simulink model "quad_with_sensor_fusion_discrete"  (R2022b)
settings: Solver=FixedStepDiscrete  StartTime=0.0  StopTime=120  FixedStep=0.005  RelTol=1e-3
values from neighbouring files (symbols this model uses):
  Ixc = 9373.661914436/1e6    (= 0.00937366191444)    [ParamsInit_test.m]
  Iyc = 11755.067703159/1e6    (= 0.0117550677032)    [ParamsInit_test.m]
  Izc = 17533.553367555/1e6    (= 0.0175335533676)    [ParamsInit_test.m]
  kd_h = damp_ratio_h*2*sqrt(kp_h*Vehicle.Airframe.mass)    [ParamsInit_test.m]
  kd_phi = damp_ratio_phi*2*sqrt(kp_phi*Ixc)    [ParamsInit_test.m]
  kd_theta = damp_ratio_theta*2*sqrt(kp_theta*Iyc)    [ParamsInit_test.m]
  kd_yaw = damp_ratio_yaw*2*sqrt(kp_yaw*Izc)    [ParamsInit_test.m]
  kp_h = omega_n_h^2*Vehicle.Airframe.mass    [ParamsInit_test.m]
  kp_phi = omega_n_phi^2*Ixc    (= 0.937366191444)    [ParamsInit_test.m]
  kp_position = 0.1    [ParamsInit_test.m]
  kp_theta = omega_n_theta^2*Iyc    (= 1.17550677032)    [ParamsInit_test.m]
  kp_vx = 0.25    [ParamsInit_test.m]
  kp_vy = 0.25    [ParamsInit_test.m]
  kp_yaw = omega_n_yaw^2*Izc    (= 0.0175335533676)    [ParamsInit_test.m]
undefined symbols (not defined in the file or in its folder): DiscIntNeverNeededParam, Vehicle
libraries: simulink x3, aerolibconvert2 x2, mspfiltlib x1, sensorinslib x1, aerolibasang x1, sharedtransform x1, mspsensorlib x1, sensorgpslib x1, aerolibanimutils x1, uavutilslib x1
(part 2 of 2)

== matlab function quad_with_sensor_fusion_discrete/Sensors and Sensor Fusion/MATLAB Function1 ==
  data: u input; y output
function y = fcn(u)

y = zeros(3,3);

a = u(1);
b = u(2);
c = u(3);

y(1,1) = cos(b)*cos(c);
y(1,2) = cos(b)*sin(c);
y(1,3) = -sin(b);
y(2,1) = sin(a)*sin(b)*cos(c)-cos(a)*sin(c);
y(2,2) = sin(a)*sin(b)*sin(c)+cos(a)*cos(c);
y(2,3) = sin(a)*cos(b);
y(3,1) = cos(a)*sin(b)*cos(c)+sin(a)*sin(c);
y(3,2) = cos(a)*sin(b)*sin(c)-sin(a)*cos(c);
y(3,3) = cos(a)*cos(b);

end

== matlab function quad_with_sensor_fusion_discrete/Plant(UAV EOM)(Non-linear)/6DOF CORE/Subsystem10/Subsystem/MATLAB Function ==
  data: m input; udot output; Fx input; V input; W input; Q input; R input
function udot = fcn(m,Fx,V,W,Q,R)
    udot = Fx/m+R*V-Q*W;
end

== matlab function quad_with_sensor_fusion_discrete/Plant(UAV EOM)(Non-linear)/6DOF CORE/Subsystem10/Subsystem1/MATLAB Function ==
  data: m input; vdot output; Fy input; U input; W input; P input; R input
function vdot = fcn(m,Fy,U,W,P,R)
    vdot = Fy/m+P*W-R*U;
end

== matlab function quad_with_sensor_fusion_discrete/Plant(UAV EOM)(Non-linear)/6DOF CORE/Subsystem10/Subsystem2/MATLAB Function ==
  data: m input; wdot output; Fz input; U input; V input; P input; Q input
function wdot = fcn(m,Fz,U,V,P,Q)
    wdot = Fz/m+Q*U-P*V;
end

== matlab function quad_with_sensor_fusion_discrete/Plant(UAV EOM)(Non-linear)/6DOF CORE/Subsystem6/MATLAB Function ==
  data: P input; phidot output; Q input; R input; phi input; theta input
function phidot = fcn(P,Q,R,phi,theta)
    phidot = P+sin(phi)*tan(theta)*Q+cos(phi)*tan(theta)*R;
end

== matlab function quad_with_sensor_fusion_discrete/Plant(UAV EOM)(Non-linear)/6DOF CORE/Subsystem6/MATLAB Function1 ==
  data: thetadot output; Q input; R input; phi input
function thetadot = fcn(Q,R,phi)
    thetadot = cos(phi)*Q-sin(phi)*R;
end

== matlab function quad_with_sensor_fusion_discrete/Outter Loop Controller/Position Control/MATLAB Function ==
  data: v input; vxr output; psi input; vyr output
function [vxr, vyr] = fcn(v,psi)
    vxr = cos(psi)*v(1)-sin(psi)*v(2);
    vyr = sin(psi)*v(1)+cos(psi)*v(2);
end

== matlab function quad_with_sensor_fusion_discrete/Plant(UAV EOM)(Non-linear)/6DOF CORE/Subsystem6/MATLAB Function2 ==
  data: pusaidot output; Q input; R input; phi input; theta input
function pusaidot = fcn(Q,R,phi,theta)
    pusaidot = sin(phi)*sec(theta)*Q+cos(phi)*sec(theta)*R;
end

== matlab function quad_with_sensor_fusion_discrete/Plant(UAV EOM)(Non-linear)/6DOF CORE/Subsystem7/Subsystem/MATLAB Function ==
  data: U input; Vxe output; V input; W input; phi input; theta input; pusai input
function Vxe = fcn(U,V,W,phi,theta,pusai)
    Vxe = cos(theta)*cos(pusai)*U+(sin(phi)*sin(theta)*cos(pusai)-cos(phi)*sin(pusai))*V+(cos(phi)*sin(theta)*cos(pusai)+sin(phi)*sin(pusai))*W;
end

== matlab function quad_with_sensor_fusion_discrete/Plant(UAV EOM)(Non-linear)/6DOF CORE/Subsystem7/Subsystem1/MATLAB Function ==
  data: U input; Vye output; V input; W input; phi input; theta input; pusai input
function Vye = fcn(U,V,W,phi,theta,pusai)
    Vye = cos(theta)*sin(pusai)*U+(sin(phi)*sin(theta)*sin(pusai)+cos(phi)*cos(pusai))*V+(cos(phi)*sin(theta)*sin(pusai)-sin(phi)*cos(pusai))*W;
end

== matlab function quad_with_sensor_fusion_discrete/Plant(UAV EOM)(Non-linear)/6DOF CORE/Subsystem7/Subsystem2/MATLAB Function ==
  data: U input; Vze output; V input; W input; phi input; theta input
function Vze = fcn(U,V,W,phi,theta)
    Vze = -sin(theta)*U+sin(phi)*cos(theta)*V+cos(phi)*cos(theta)*W;
end

== matlab function quad_with_sensor_fusion_discrete/Plant(UAV EOM)(Non-linear)/6DOF CORE/Subsystem8/MATLAB Function ==
  data: u input; y output
function y = fcn(u)

y = zeros(3,3);

a = u(1);
b = u(2);
c = u(3);

y(1,1) = cos(b)*cos(c);
y(1,2) = cos(b)*sin(c);
y(1,3) = -sin(b);
y(2,1) = sin(a)*sin(b)*cos(c)-cos(a)*sin(c);
y(2,2) = sin(a)*sin(b)*sin(c)+cos(a)*cos(c);
y(2,3) = sin(a)*cos(b);
y(3,1) = cos(a)*sin(b)*cos(c)+sin(a)*sin(c);
y(3,2) = cos(a)*sin(b)*sin(c)-sin(a)*cos(c);
y(3,3) = cos(a)*cos(b);

end

== matlab function quad_with_sensor_fusion_discrete/Inner Loop Controller/ToRPM ==
  data: tau_x input; omega_square output; tau_y input; tau_z input; T input
function omega_square = fcn(tau_x,tau_y,tau_z,T)
    input = [tau_x;tau_y;tau_z;T];
    diameter = 0.410;
    k_tau = 1.779e-7;
    k_T = 1.097e-5;
    k = diameter/2*k_tau/sqrt(2);
    A = [-k k k -k;
        k -k k -k;
        -k_tau -k_tau k_tau k_tau;
        -k_T -k_T -k_T -k_T];
    omega_square = A\input;
end

== matlab function quad_with_sensor_fusion_discrete/Plant(UAV EOM)(Non-linear)/6DOF CORE/Subsystem/MATLAB Function ==
  data: I input; P_dot output; M input size=[3,1]; omega input size=[3,1]; Q_dot output; R_dot output
function [P_dot, Q_dot, R_dot] = fcn(I,M,omega)
    omega_dot = M-cross(omega,(I*omega));
    P_dot = omega_dot(1)/I(1,1);
    Q_dot = omega_dot(2)/I(2,2);
    R_dot = omega_dot(3)/I(3,3);
end

== matlab function quad_with_sensor_fusion_discrete/Actuator(Motors)1/Propeller Model ==
  data: Mb_xy output; F input; R input
function Mb_xy  = fcn(F,R)
 %%叉字型
 %3  1
 %2  4
 M_rctcm = [-sin(pi/4)*R,sin(pi/4)*R,sin(pi/4)*R,-sin(pi/4)*R;
            sin(pi/4)*R,-sin(pi/4)*R,sin(pi/4)*R,-sin(pi/4)*R];
 Mb_xy = M_rctcm*(F);%式(6.24),力矩

end

== matlab function quad_with_sensor_fusion_discrete/Sensors and Sensor Fusion/MATLAB Function ==
  data: t input; y output
function y = fcn(t)
    if(abs(t-(round(t))))<=1e-3
        y = 1;
    else
        y = 0;
    end
end

== matlab function quad_with_sensor_fusion_discrete/Actuator(Motors)/Propeller Model ==
  data: Mb_xy output; F input
function Mb_xy  = fcn(F)
 %%叉字型
 %3  1
 %2  4
 R = 0.205;
 M_rctcm = [-sin(pi/4)*R,sin(pi/4)*R,sin(pi/4)*R,-sin(pi/4)*R;
            sin(pi/4)*R,-sin(pi/4)*R,sin(pi/4)*R,-sin(pi/4)*R;
            -1,-1,1,1];
 Mb_xy = M_rctcm*(F);%式(6.24),力矩

end

== matlab function quad_with_sensor_fusion_discrete/Sensors and Sensor Fusion/Subsystem6/MATLAB Function ==
  data: P input; phidot output; Q input; R input; phi input; theta input
function phidot = fcn(P,Q,R,phi,theta)
    phidot = P+sin(phi)*tan(theta)*Q+cos(phi)*tan(theta)*R;
end

== matlab function quad_with_sensor_fusion_discrete/Sensors and Sensor Fusion/Subsystem6/MATLAB Function1 ==
  data: thetadot output; Q input; R input; phi input
function thetadot = fcn(Q,R,phi)
    thetadot = cos(phi)*Q-sin(phi)*R;
end

== matlab function quad_with_sensor_fusion_discrete/Sensors and Sensor Fusion/Subsystem6/MATLAB Function2 ==
  data: pusaidot output; Q input; R input; phi input; theta input
function pusaidot = fcn(Q,R,phi,theta)
    pusaidot = sin(phi)*sec(theta)*Q+cos(phi)*sec(theta)*R;
end
